simulink model "MPPT_2022b_new"  (R2022b)
settings: Solver=VariableStepAuto  StartTime=0.0  StopTime=0.5  RelTol=1e-3
libraries: spsVariableCapacitorLib x4, spsCurrentMeasurementLib x3, spsDiodeLib x3, spsMosfetLib x3, spsVoltageMeasurementLib x3, spsVariableInductorLib x2, spsVariableResistorLib x2, slpidlib x1, simulink x1, spsPVArrayLib x1, spsPWMGeneratorDCDCLib x1, spspowerguiLib x1
settings Model: Creator=Riley  LastModifiedBy=user
settings OptimizationCC: ReuseModelBlockBuffer=on

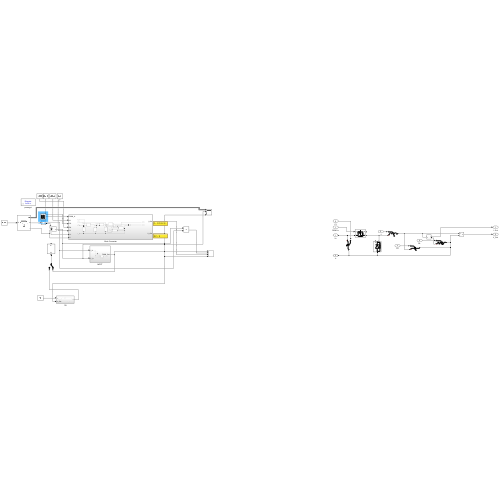
[thumbnail: Simulink's stored preview of the top-level diagram]
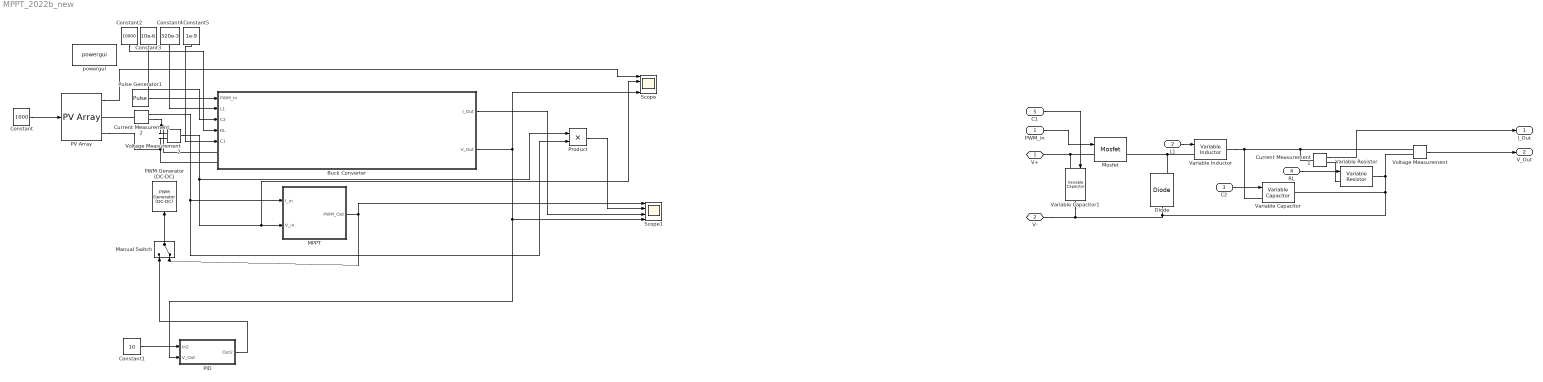
== system MPPT_2022b_new ==
  PWM_in : Inport
  L1 : Inport  Port=2
  C2 : Inport  Port=3
  RL : Inport  Port=4
  C1 : Inport  Port=5
  Buck Converter : Subsystem
  Constant : Constant  Value=1000
  Constant1 : Constant  Value=10
  Constant2 : Constant  Value=10000
  Constant3 : Constant  Value=10e-6
  Constant4 : Constant  Value=320e-3
  Constant5 : Constant  Value=1e-9
  Current Measurement1 : spsCurrentMeasurementLib/Current Measurement  PhasorSimulation=off  OutputType=Complex  PSBequivalent=0
  Current Measurement2 : spsCurrentMeasurementLib/Current Measurement  PhasorSimulation=off  OutputType=Complex  PSBequivalent=0
  Diode : spsDiodeLib/Diode  Ron=0.001  Lon=0  Vf=0.8  IC=0  UseSnubber=0  Rs=500  Cs=250e-9  Measurements=on
  MPPT : Subsystem
  Manual Switch : ManualSwitch  CurrentSetting=0
  Mosfet : spsMosfetLib/Mosfet  Ron=3.2e-3  Lon=0  Rd=1e-6  Vfd=0  IC=0  Rs=1e5  Cs=inf  Measurements=on
  PID : Subsystem
  PV Array : spsPVArrayLib/PV Array  Npar=1  Nser=1  PlotType=array @ 1000 W/m2 & specified temperatures  S_vec="[ 1000  500  100 ]"  Temp_C_vec="[ 45 25  ]"  ModuleName=User-defined  PlotWhenSelected=off  Pm=10.208  Ncell=60  Voc=22.0  Isc=0.60  Vm=17.6  Im=0.58  beta_Voc_pc=-0.36  alpha_Isc_pc=0.10  beta_Voc=-0.0792  alpha_Isc=0.0006  IL=0.61105  I0=2.15e-11  nI=0.59304  Rsh=6907.0501  Rs=3.0088  RobustModel=on  RobustCellTemperature=25  BAL=on  Tc=1e-6  Tfilter=5e-5
  PWM Generator (DC-DC) : spsPWMGeneratorDCDCLib/PWM Generator (DC-DC)  Fsw=39000  Ts=1e-6
  Product : Product
  Pulse Generator1 : DiscretePulseGenerator  PulseType=Time based  Amplitude=5  Period=1/32000  PulseWidth=80
  Scope : Scope  NumInputPorts=4
  Scope1 : Scope  NumInputPorts=4
  Variable Capacitor : spsVariableCapacitorLib/Variable Capacitor  methode=Backward Euler  Cabsmin=1e-9  Initialize=off  vC0=0  C0=1e-6  iC0=0
      settings: LibrarySourceBlock=sps_lib/Passives/Variable Capacitor
  Variable Capacitor1 : spsVariableCapacitorLib/Variable Capacitor  methode=Backward Euler  Cabsmin=1e-9  Initialize=off  vC0=0  C0=1e-6  iC0=0
      settings: LibrarySourceBlock=sps_lib/Passives/Variable Capacitor
  Variable Inductor : spsVariableInductorLib/Variable Inductor  methode=Backward Euler  Labsmin=1e-6  Initialize=off  iL0=0  L0=1e-3  Vl0=0
      settings: LibrarySourceBlock=sps_lib/Passives/Variable Inductor
  Variable Resistor : spsVariableResistorLib/Variable Resistor  Rabsmin=1e-3
      settings: LibrarySourceBlock=sps_lib/Passives/Variable Resistor
  Voltage Measurement : spsVoltageMeasurementLib/Voltage Measurement  PhasorSimulation=off  OutputType=Complex  PSBequivalent=0
  Voltage Measurement2 : spsVoltageMeasurementLib/Voltage Measurement  PhasorSimulation=off  OutputType=Complex  PSBequivalent=0
  powergui : spspowerguiLib/powergui  Priority=1  SimulationMode=Discrete  SampleTime=1e-6  frequency=60  Iterations=50  frequencyindice=0  Pbase=100e6  ErrMax=1e-4  UnitsV=kV  UnitsW=MW  buscounter=0  FunctionMessages=off  echomessages=off  EnableUseOfTLC=off  CurrentSourceSwitches=off  DisableSnubberDevices=off  DisableRonSwitches=off  DisableVfSwitches=off  DisplayEquations=off  AutomaticDiscreteSolvers=off  SolverType=Tustin/Backward Euler (TBE)  Interpol=off  ExternalGateDelay=off  methode=off  Ts=100  x0status=blocks  SPID=on  SwTol=0  HookPort=off  NonlinearTolerance=1e-4  nMaxIteration=100  ContinueOnMaxIteration=on  RestoreLinks=warning  ResistiveCurrentMeasurement=off  Frange=[0:2:500]  Ylog=off  Xlog=on  ShowGrid=off  save=off  variable=ZData  structure=0  ZoomFFT=off  StartTime=0.0  cycles=1  DisplayStyle=1  fundamental=60  FreqAxis=off  MaxFrequency=1000  frequencyindicesteady=1  RmsSteady=1  display=off
  V+ : PMIOPort  Side=Left
  V- : PMIOPort  Port=2  Side=Left
  I_Out : Outport
  V_Out : Outport  Port=2
  wires:
  Constant/1 -> PV Array/1
  PV Array/1 -> Scope/1
  PID/1(Out2) -> Manual Switch/1
  Constant1/1 -> PID/1(In2)
  Buck Converter/2(V_Out) -> Scope/4, Scope1/4, PID/2(V_Out)
  Buck Converter/1(I_Out) -> Scope1/3
  Manual Switch/1 -> PWM Generator (DC-DC)/1
  MPPT/1(PWM_Out) -> Scope1/1, Manual Switch/2
  Current Measurement2/1 -> Product/2, MPPT/1(I_in)
  Voltage Measurement2/1 -> Product/1, Scope/2, MPPT/2(V_in)
  Constant4/1 -> Buck Converter/2(L1)
  Constant3/1 -> Buck Converter/3(C2)
  Constant2/1 -> Buck Converter/4(RL)
  Product/1 -> Scope1/2
  Constant5/1 -> Buck Converter/5(C1)
  L1/1 -> Variable Inductor/1
  Voltage Measurement/1 -> V_Out/1
  Current Measurement1/1 -> I_Out/1
  PWM_in/1 -> Mosfet/1
  C2/1 -> Variable Capacitor/1
  C1/1 -> Variable Capacitor1/1
  RL/1 -> Variable Resistor/1
  Pulse Generator1/1 -> Buck Converter/1(PWM_in)
  connections:
  Voltage Measurement2/LConn1 -- Buck Converter/LConn1 -- Current Measurement2/RConn1
  PV Array/RConn2 -- Buck Converter/LConn2 -- Voltage Measurement2/LConn2
  Current Measurement2/LConn1 -- PV Array/RConn1
  Variable Capacitor1/LConn1 -- V+/RConn1 -- Mosfet/LConn1
  Diode/LConn1 -- Voltage Measurement/LConn2 -- Variable Resistor/RConn1 -- Variable Capacitor/RConn1 -- V-/RConn1 -- Variable Capacitor1/RConn1
  Voltage Measurement/LConn1 -- Variable Inductor/RConn1 -- Variable Capacitor/LConn1 -- Current Measurement1/LConn1
  Diode/RConn1 -- Mosfet/RConn1 -- Variable Inductor/LConn1
  Current Measurement1/RConn1 -- Variable Resistor/LConn1

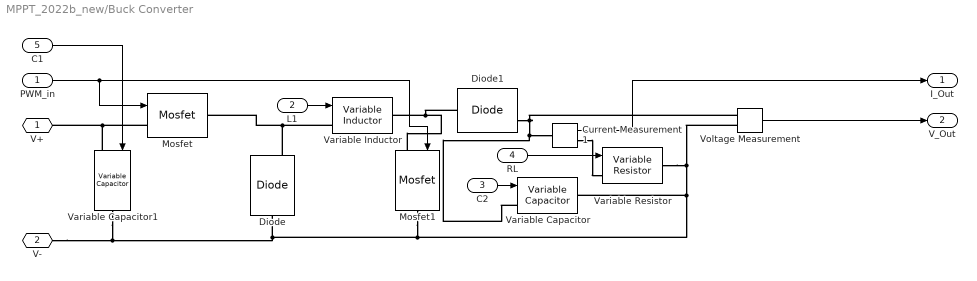
== system MPPT_2022b_new/Buck Converter ==
  PWM_in : Inport
  L1 : Inport  Port=2
  C2 : Inport  Port=3
  RL : Inport  Port=4
  C1 : Inport  Port=5
  Current Measurement1 : spsCurrentMeasurementLib/Current Measurement  PhasorSimulation=off  OutputType=Complex  PSBequivalent=0
  Diode : spsDiodeLib/Diode  Ron=0.001  Lon=0  Vf=0.8  IC=0  UseSnubber=0  Rs=500  Cs=250e-9  Measurements=on
  Diode1 : spsDiodeLib/Diode  Ron=0.001  Lon=0  Vf=0.8  IC=0  UseSnubber=0  Rs=500  Cs=250e-9  Measurements=on
  Mosfet : spsMosfetLib/Mosfet  Ron=3.2e-3  Lon=0  Rd=1e-6  Vfd=0  IC=0  Rs=1e5  Cs=inf  Measurements=off
  Mosfet1 : spsMosfetLib/Mosfet  Ron=3.2e-3  Lon=0  Rd=1e-6  Vfd=0  IC=0  Rs=1e5  Cs=inf  Measurements=off
  Variable Capacitor : spsVariableCapacitorLib/Variable Capacitor  methode=Backward Euler  Cabsmin=1e-9  Initialize=off  vC0=0  C0=1e-6  iC0=0
      settings: LibrarySourceBlock=sps_lib/Passives/Variable Capacitor
  Variable Capacitor1 : spsVariableCapacitorLib/Variable Capacitor  methode=Backward Euler  Cabsmin=1e-9  Initialize=off  vC0=0  C0=1e-6  iC0=0
      settings: LibrarySourceBlock=sps_lib/Passives/Variable Capacitor
  Variable Inductor : spsVariableInductorLib/Variable Inductor  methode=Backward Euler  Labsmin=1e-6  Initialize=off  iL0=0  L0=1e-3  Vl0=0
      settings: LibrarySourceBlock=sps_lib/Passives/Variable Inductor
  Variable Resistor : spsVariableResistorLib/Variable Resistor  Rabsmin=1e-3
      settings: LibrarySourceBlock=sps_lib/Passives/Variable Resistor
  Voltage Measurement : spsVoltageMeasurementLib/Voltage Measurement  PhasorSimulation=off  OutputType=Complex  PSBequivalent=0
  V+ : PMIOPort  Side=Left
  V- : PMIOPort  Port=2  Side=Left
  I_Out : Outport
  V_Out : Outport  Port=2
  wires:
  Current Measurement1/1 -> I_Out/1
  C2/1 -> Variable Capacitor/1
  RL/1 -> Variable Resistor/1
  L1/1 -> Variable Inductor/1
  Voltage Measurement/1 -> V_Out/1
  PWM_in/1 -> Mosfet1/1, Mosfet/1
  C1/1 -> Variable Capacitor1/1
  connections:
  Diode/LConn1 -- Mosfet1/RConn1 -- Voltage Measurement/LConn2 -- Variable Resistor/RConn1 -- Variable Capacitor/RConn1 -- V-/RConn1 -- Variable Capacitor1/RConn1
  Voltage Measurement/LConn1 -- Diode1/RConn1 -- Variable Capacitor/LConn1 -- Current Measurement1/LConn1
  Diode/RConn1 -- Mosfet/RConn1 -- Variable Inductor/LConn1
  V+/RConn1 -- Mosfet/LConn1 -- Variable Capacitor1/LConn1
  Current Measurement1/RConn1 -- Variable Resistor/LConn1
  Diode1/LConn1 -- Variable Inductor/RConn1 -- Mosfet1/LConn1

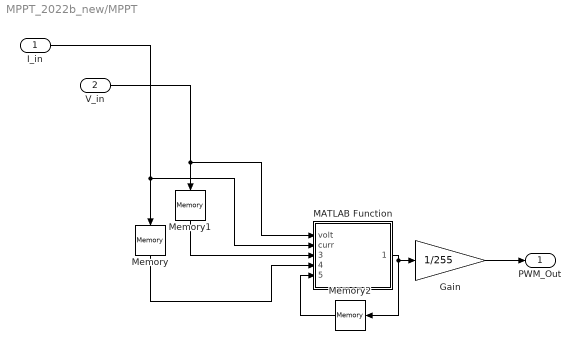
== system MPPT_2022b_new/MPPT ==
  I_in : Inport
  V_in : Inport  Port=2
  Gain : Gain  Gain=1/255
  MATLAB Function : MATLAB Function  TreatAsAtomicUnit=on
  Memory : Memory  InheritSampleTime=on
  Memory1 : Memory  InheritSampleTime=on
  Memory2 : Memory  InheritSampleTime=on
  PWM_Out : Outport
  wires:
  I_in/1 -> Memory/1, MATLAB Function/2(curr)
  Memory1/1 -> MATLAB Function/3(volt_prev)
  MATLAB Function/1(pwm_out) -> Memory2/1, Gain/1
  Memory2/1 -> MATLAB Function/5(pwm_in)
  V_in/1 -> Memory1/1, MATLAB Function/1(volt)
  Memory/1 -> MATLAB Function/4(curr_prev)
  Gain/1 -> PWM_Out/1

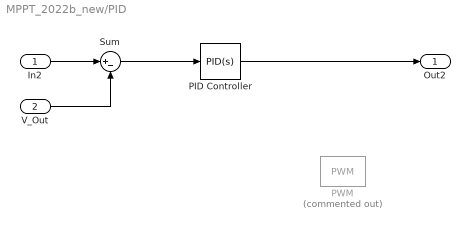
== system MPPT_2022b_new/PID ==
  In2 : Inport
  V_Out : Inport  Port=2
  PID Controller : slpidlib/PID Controller  Controller=PID  Form=Parallel  TimeDomain=Continuous-time  UseExternalTs=off  SampleTime=-1  IntegratorMethod=Forward Euler  FilterMethod=Forward Euler  ControllerParametersSource=internal  P=2  I=1  UseKiTs=off  D=0  N=100  UseFilter=on  TunerSelectOption=Transfer Function Based (PID Tuner App)  InitialConditionSource=internal  InitialConditionForIntegrator=0  InitialConditionForFilter=0  DifferentiatorICPrevScaledInput=0  ExternalReset=none  TrackingMode=off  Kt=1  LimitOutput=off  SatLimitsSource=internal  UpperSaturationLimit=inf  LowerSaturationLimit=-inf  LinearizeAsGain=on  AntiWindupMode=none  Kb=1  LimitIntegrator=off  UpperIntegratorSaturationLimit=inf  LowerIntegratorSaturationLimit=-inf  POutMin=[]  POutMax=[]  IOutMin=[]  IOutMax=[]  DOutMin=[]  DOutMax=[]  NOutMin=[]  NOutMax=[]  SumOutMin=[]  SumOutMax=[]  SaturationOutMin=[]  SaturationOutMax=[]  PParamMin=[]  PParamMax=[]  IParamMin=[]  IParamMax=[]  DParamMin=[]  DParamMax=[]  NParamMin=[]  NParamMax=[]  KbParamMin=[]  KbParamMax=[]  KtParamMin=[]  KtParamMax=[]  KbOutMin=[]  KbOutMax=[]  KtOutMin=[]  KtOutMax=[]  IntegratorOutMin=[]  IntegratorOutMax=[]  FilterOutMin=[]  FilterOutMax=[]  SumI1OutMin=[]  SumI1OutMax=[]  SumI2OutMin=[]  SumI2OutMax=[]  SumI3OutMin=[]  SumI3OutMax=[]  SumI4OutMin=[]  SumI4OutMax=[]  SumDOutMin=[]  SumDOutMax=[]  DifferentiatorOutMin=[]  DifferentiatorOutMax=[]  FilterDiffOutCoefMin=[]  FilterDiffOutCoefMax=[]  ReciprocalOutMin=[]  ReciprocalOutMax=[]  SumDenOutMin=[]  SumDenOutMax=[]  SumNumOutMin=[]  SumNumOutMax=[]  DivideOutMin=[]  DivideOutMax=[]  UdiffTsProdOutMin=[]  UdiffTsProdOutMax=[]  NTsProdOutMin=[]  NTsProdOutMax=[]  UintegralTsProdOutMin=[]  UintegralTsProdOutMax=[]  UngainTsProdOutMin=[]  UngainTsProdOutMax=[]  ClampingZeroOutDataTypeStr=Inherit: Inherit via back propagation  ClampingZeroOutMin=[]  ClampingZeroOutMax=[]  FilterDenConstantOutDataTypeStr=Inherit: Inherit via back propagation  FilterDenConstantOutMin=[]  FilterDenConstantOutMax=[]  PCopyOutDataTypeStr=Inherit: Inherit via back propagation  PCopyOutMin=[]  PCopyOutMax=[]  NCopyOutDataTypeStr=Inherit: Inherit via back propagation  NCopyOutMin=[]  NCopyOutMax=[]  IntegratorContinuousStateAttributes=''  IntegratorStateMustResolveToSignalObject=off  IntegratorRTWStateStorageClass=Auto  FilterContinuousStateAttributes=''  FilterStateMustResolveToSignalObject=off  FilterRTWStateStorageClass=Auto  ParallelPVariant=InternalParameters  IdealPVariant=Disabled  IVariant=InternalParameters  DVariant=InternalParameters  IntegratorVariant=Continuous  SatVariant=Disabled  AWVariant=Passthrough  PCopyVariant=Disabled  TRVariant=Disabled  FdbkBlocksVariant=Forward  IdealPFdbkVariant=Disabled  SatFdbkVariant=Disabled  DerivativeFilterVariant=ContFilter  NVariant=InternalParameters  NCopyVariant=Disabled  FilterICVariant=InternalICsFilter  IntegratorICVariant=InternalICs  ExternalResetVariant=Disabled  TRSumVariant=Passthrough  SumFdbkVariant=Disabled  SumVariant=Sum_PID  TsampFilterVariant=InternalTs  TsampNgainVariant=Passthrough  TsampIntegralVariant=Passthrough  ExternalSaturationOutDataTypeStr=Inherit: Same as second input
  PWM : simulink/Discontinuities/PWM  Commented=on  DisableCoverage=on  Period=1e-5  InitialDelay=0  DisallowZeroDutyCycle=off  RunAtFixedTimeIntervals=off  SampleTime=0.1
  Sum : Sum  Inputs=|+-
  Out2 : Outport
  wires:
  In2/1 -> Sum/1
  Sum/1 -> PID Controller/1
  V_Out/1 -> Sum/2
  PID Controller/1 -> Out2/1

== matlab function MPPT_2022b_new/MPPT/MATLAB Function ==
  data: volt input; pwm_out output; curr input; volt_prev input; curr_prev input; pwm_in input
function pwm_out = fcn(volt, curr, volt_prev, curr_prev, pwm_in)

% Code to update the PWM voltage
delta_v = volt - volt_prev;
delta_i = curr - curr_prev;

delta_const = curr + (delta_i/delta_v)*volt;

if delta_v == 0
    if delta_i == 0
        pwm_out = pwm_in;
    elseif delta_i > 0
        pwm_out = pwm_in + 1;
    else
        pwm_out = pwm_in - 1;
    end
elseif delta_const == 0
    pwm_out = pwm_in + 1;
elseif delta_const > 0
    pwm_out = pwm_in + 1;
else
    pwm_out = pwm_in - 1;
end

% Saturating output
if pwm_out > 250
    pwm_out = 250;
elseif pwm_out < 5
    pwm_out = 5;
end
